simulink model "Four_PureSine_3Ph_Inv"  (R2024a)
settings: Solver=VariableStepAuto  StartTime=0.0  StopTime=0.3  RelTol=1e-6
libraries: spsSeriesRLCBranchLib x9, spsIGBTLib x6, spsSawtoothGeneratorLib x3, spsGroundLib x2, spsThreePhaseVIMeasurementLib x2, spsDCVoltageSourceLib x1, sps_lib x1
settings Model: Creator=91889  LastModifiedBy=91889

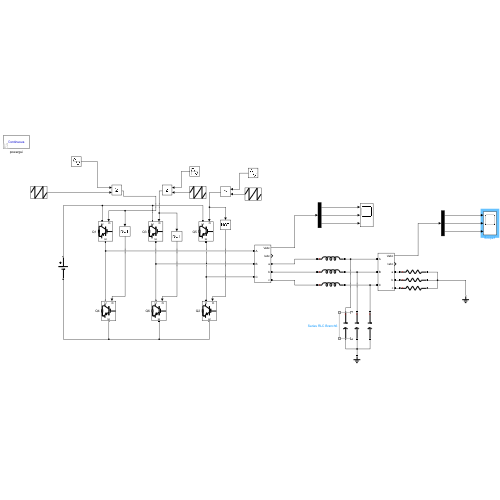
[thumbnail: Simulink's stored preview of the top-level diagram]
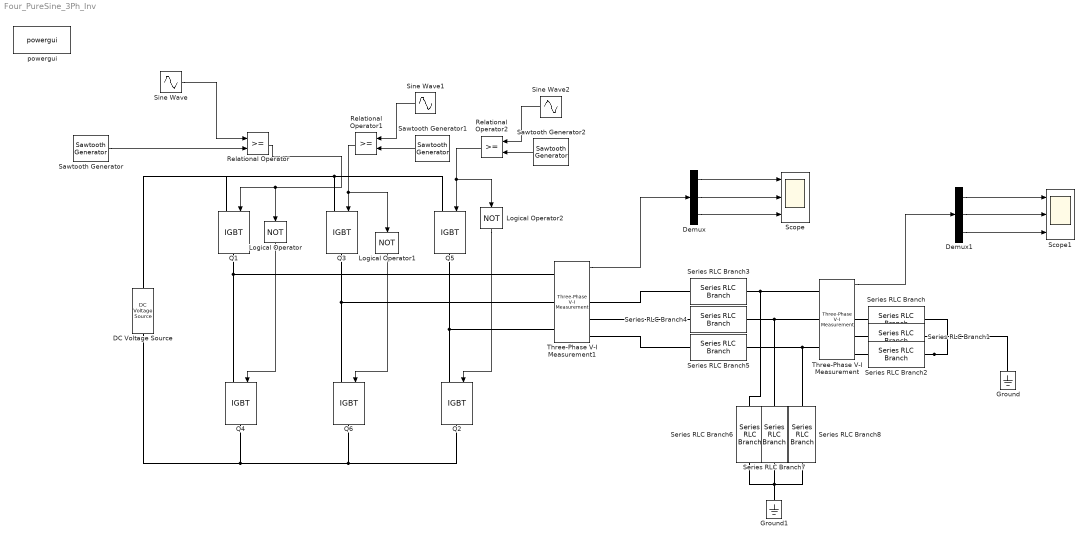
== system Four_PureSine_3Ph_Inv ==
  DC Voltage Source : spsDCVoltageSourceLib/DC Voltage Source  Amplitude=100  Measurements=None
  Demux : Demux  Outputs=3
  Demux1 : Demux  Outputs=3
  Ground : spsGroundLib/Ground  LConnTagsString=a
  Ground1 : spsGroundLib/Ground  LConnTagsString=a
  Logical Operator : Logic  Operator=NOT  AllPortsSameDT=off  OutDataTypeStr=boolean
  Logical Operator1 : Logic  Operator=NOT  AllPortsSameDT=off  OutDataTypeStr=boolean
  Logical Operator2 : Logic  Operator=NOT  AllPortsSameDT=off  OutDataTypeStr=boolean
  Q{1..6} (6 alike) : spsIGBTLib/IGBT  Ron=0.001  Lon=0  Vf=1  Tf=1e-6  Tt=2e-6  IC=0  Rs=1e5  Cs=inf  Measurements=off
  Relational Operator : RelationalOperator  OutDataTypeStr=boolean  RndMeth=Simplest  InputSameDT=off
  Relational Operator1 : RelationalOperator  OutDataTypeStr=boolean  RndMeth=Simplest  InputSameDT=off
  Relational Operator2 : RelationalOperator  OutDataTypeStr=boolean  RndMeth=Simplest  InputSameDT=off
  Sawtooth Generator : spsSawtoothGeneratorLib/Sawtooth Generator  Freq=750  Phase=180  Ts=0
  Sawtooth Generator1 : spsSawtoothGeneratorLib/Sawtooth Generator  Freq=750  Phase=180  Ts=0
  Sawtooth Generator2 : spsSawtoothGeneratorLib/Sawtooth Generator  Freq=750  Phase=180  Ts=0
  Scope : Scope  NumInputPorts=3
  Scope1 : Scope  NumInputPorts=3
  Series RLC Branch : spsSeriesRLCBranchLib/Series RLC Branch  LConnTagsString=__new0  RConnTagsString=__new0  BranchType=R  Resistance=30  Inductance=1e-3  SetiL0=off  InitialCurrent=0  Capacitance=1e-6  Setx0=off  InitialVoltage=0  Measurements=None
  Series RLC Branch1 : spsSeriesRLCBranchLib/Series RLC Branch  LConnTagsString=__new0  RConnTagsString=__new0  BranchType=R  Resistance=30  Inductance=1e-3  SetiL0=off  InitialCurrent=0  Capacitance=1e-6  Setx0=off  InitialVoltage=0  Measurements=None
  Series RLC Branch2 : spsSeriesRLCBranchLib/Series RLC Branch  LConnTagsString=__new0  RConnTagsString=__new0  BranchType=R  Resistance=30  Inductance=1e-3  SetiL0=off  InitialCurrent=0  Capacitance=1e-6  Setx0=off  InitialVoltage=0  Measurements=None
  Series RLC Branch3 : spsSeriesRLCBranchLib/Series RLC Branch  LConnTagsString=__new0  RConnTagsString=__new0  BranchType=L  Resistance=10  Inductance=100e-3  SetiL0=off  InitialCurrent=0  Capacitance=1e-6  Setx0=off  InitialVoltage=0  Measurements=None
  Series RLC Branch4 : spsSeriesRLCBranchLib/Series RLC Branch  LConnTagsString=__new0  RConnTagsString=__new0  BranchType=L  Resistance=10  Inductance=100e-3  SetiL0=off  InitialCurrent=0  Capacitance=1e-6  Setx0=off  InitialVoltage=0  Measurements=None
  Series RLC Branch5 : spsSeriesRLCBranchLib/Series RLC Branch  LConnTagsString=__new0  RConnTagsString=__new0  BranchType=L  Resistance=10  Inductance=100e-3  SetiL0=off  InitialCurrent=0  Capacitance=1e-6  Setx0=off  InitialVoltage=0  Measurements=None
  Series RLC Branch6 : spsSeriesRLCBranchLib/Series RLC Branch  LConnTagsString=__new0  RConnTagsString=__new0  BranchType=C  Resistance=10  Inductance=80e-3  SetiL0=off  InitialCurrent=0  Capacitance=300e-6  Setx0=off  InitialVoltage=0  Measurements=None
  Series RLC Branch7 : spsSeriesRLCBranchLib/Series RLC Branch  LConnTagsString=__new0  RConnTagsString=__new0  BranchType=C  Resistance=10  Inductance=80e-3  SetiL0=off  InitialCurrent=0  Capacitance=300e-6  Setx0=off  InitialVoltage=0  Measurements=None
  Series RLC Branch8 : spsSeriesRLCBranchLib/Series RLC Branch  LConnTagsString=__new0  RConnTagsString=__new0  BranchType=C  Resistance=10  Inductance=80e-3  SetiL0=off  InitialCurrent=0  Capacitance=300e-6  Setx0=off  InitialVoltage=0  Measurements=None
  Sine Wave : Sin  Amplitude=0.9  Frequency=2*pi*50  SampleTime=0
  Sine Wave1 : Sin  Amplitude=0.9  Frequency=2*pi*50  Phase=120*(pi/180)  SampleTime=0
  Sine Wave2 : Sin  Amplitude=0.9  Frequency=2*pi*50  Phase=240*(pi/180)  SampleTime=0
  Three-Phase V-I Measurement : spsThreePhaseVIMeasurementLib/Three-Phase V-I Measurement  VoltageMeasurement=phase-to-phase  SetLabelV=off  LabelV=Vabc  Vpu=off  VpuLL=off  CurrentMeasurement=yes  SetLabelI=off  LabelI=Iabc  Ipu=off  Pbase=100e6  Vbase=500e3  OutputType=Complex  PhasorSimulation=off  PSBequivalent=0
  Three-Phase V-I Measurement1 : spsThreePhaseVIMeasurementLib/Three-Phase V-I Measurement  VoltageMeasurement=phase-to-phase  SetLabelV=off  LabelV=Vabc  Vpu=off  VpuLL=off  CurrentMeasurement=yes  SetLabelI=off  LabelI=Iabc  Ipu=off  Pbase=100e6  Vbase=500e3  OutputType=Complex  PhasorSimulation=off  PSBequivalent=0
  powergui : sps_lib/powergui  Priority=1  SimulationMode=Continuous  SampleTime=50e-6  frequency=60  Iterations=50  frequencyindice=0  Pbase=100e6  ErrMax=1e-4  UnitsV=kV  UnitsW=MW  buscounter=0  FunctionMessages=off  echomessages=off  EnableUseOfTLC=off  CurrentSourceSwitches=off  DisableSnubberDevices=off  DisableRonSwitches=off  DisableVfSwitches=off  DisplayEquations=off  AutomaticDiscreteSolvers=off  SolverType=Tustin/Backward Euler (TBE)  Interpol=off  ExternalGateDelay=off  methode=off  Ts=100  x0status=blocks  SPID=on  SwTol=0  HookPort=off  NonlinearTolerance=1e-4  nMaxIteration=100  ContinueOnMaxIteration=off  RestoreLinks=warning  ResistiveCurrentMeasurement=off  Frange=[0:2:500]  Ylog=off  Xlog=on  ShowGrid=off  save=off  variable=ZData  structure=0  ZoomFFT=off  StartTime=0.0  cycles=1  DisplayStyle=1  fundamental=60  FreqAxis=off  MaxFrequency=1000  frequencyindicesteady=1  RmsSteady=1  display=off
  wires:
  Logical Operator2/1 -> Q2/1
  Demux/1 -> Scope/1
  Sine Wave/1 -> Relational Operator/1
  Demux/2 -> Scope/2
  Logical Operator/1 -> Q4/1
  Sawtooth Generator1/1 -> Relational Operator1/2
  Sine Wave2/1 -> Relational Operator2/1
  Sawtooth Generator2/1 -> Relational Operator2/2
  Logical Operator1/1 -> Q6/1
  Sine Wave1/1 -> Relational Operator1/1
  Relational Operator1/1 -> Logical Operator1/1, Q3/1
  Demux/3 -> Scope/3
  Relational Operator2/1 -> Logical Operator2/1, Q5/1
  Relational Operator/1 -> Q1/1, Logical Operator/1
  Sawtooth Generator/1 -> Relational Operator/2
  Three-Phase V-I Measurement1/1 -> Demux/1
  Three-Phase V-I Measurement/1 -> Demux1/1
  Demux1/3 -> Scope1/3
  Demux1/2 -> Scope1/2
  Demux1/1 -> Scope1/1
  connections:
  DC Voltage Source/LConn1 -- Q4/RConn1 -- Q6/RConn1 -- Q2/RConn1
  Q3/LConn1 -- Q5/LConn1 -- Q1/LConn1 -- DC Voltage Source/RConn1
  Q5/RConn1 -- Q2/LConn1 -- Three-Phase V-I Measurement1/LConn3
  Q1/RConn1 -- Three-Phase V-I Measurement1/LConn1 -- Q4/LConn1
  Q3/RConn1 -- Q6/LConn1 -- Three-Phase V-I Measurement1/LConn2
  Series RLC Branch2/RConn1 -- Series RLC Branch/RConn1 -- Ground/LConn1 -- Series RLC Branch1/RConn1
  Three-Phase V-I Measurement/RConn3 -- Series RLC Branch2/LConn1
  Three-Phase V-I Measurement/RConn1 -- Series RLC Branch/LConn1
  Three-Phase V-I Measurement/RConn2 -- Series RLC Branch1/LConn1
  Series RLC Branch3/RConn1 -- Series RLC Branch6/LConn1 -- Three-Phase V-I Measurement/LConn1
  Series RLC Branch4/RConn1 -- Three-Phase V-I Measurement/LConn2 -- Series RLC Branch7/LConn1
  Series RLC Branch5/RConn1 -- Three-Phase V-I Measurement/LConn3 -- Series RLC Branch8/LConn1
  Three-Phase V-I Measurement1/RConn1 -- Series RLC Branch3/LConn1
  Three-Phase V-I Measurement1/RConn2 -- Series RLC Branch4/LConn1
  Three-Phase V-I Measurement1/RConn3 -- Series RLC Branch5/LConn1
  Series RLC Branch6/RConn1 -- Series RLC Branch8/RConn1 -- Series RLC Branch7/RConn1 -- Ground1/LConn1
